simulink model "House_model"  (R2016b)
settings: Solver=VariableStepAuto  StartTime=0.0  StopTime=inf  RelTol=1e-3
settings Model: Creator=isabelle  LastModifiedBy=Josefine

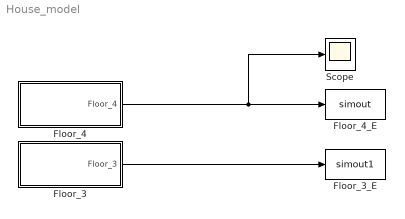
== system House_model ==
  Floor_3 : Subsystem
  Floor_3_E : ToWorkspace  VariableName=simout1  SaveFormat=Timeseries  SampleTime=-1
  Floor_4 : Subsystem
  Floor_4_E : ToWorkspace  VariableName=simout  SaveFormat=Timeseries  SampleTime=-1
  Scope : Scope
  wires:
  Floor_4/1(Floor_4) -> Scope/1, Floor_4_E/1
  Floor_3/1(Floor_3) -> Floor_3_E/1

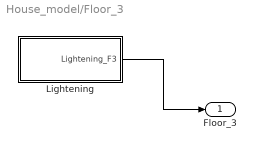
== system House_model/Floor_3 ==
  Lightening : Subsystem
  Floor_3 : Outport
  wires:
  Lightening/1(Lightening_F3) -> Floor_3/1

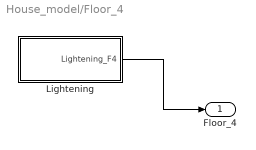
== system House_model/Floor_4 ==
  Lightening : Subsystem
  Floor_4 : Outport
  wires:
  Lightening/1(Lightening_F4) -> Floor_4/1

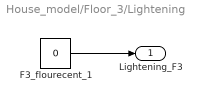
== system House_model/Floor_3/Lightening ==
  F3_flourecent_1 : Constant  Value=0
  Lightening_F3 : Outport
  wires:
  F3_flourecent_1/1 -> Lightening_F3/1

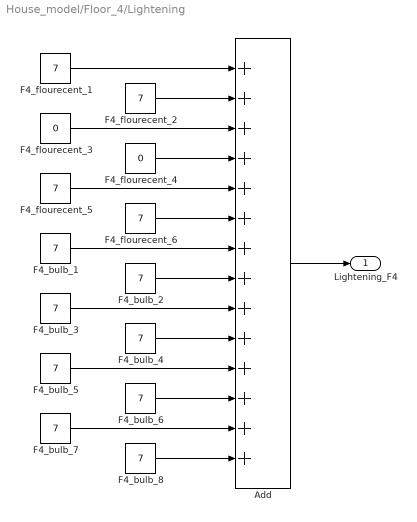
== system House_model/Floor_4/Lightening ==
  Add : Sum  Inputs=14
  F4_bulb_{1..8} (8 alike) : Constant  Value=7
  F4_flourecent_{1..2,5..6} (4 alike) : Constant  Value=7
  F4_flourecent_3 : Constant  Value=0
  F4_flourecent_4 : Constant  Value=0
  Lightening_F4 : Outport
  wires:
  F4_flourecent_1/1 -> Add/1
  F4_flourecent_2/1 -> Add/2
  F4_flourecent_3/1 -> Add/3
  F4_flourecent_4/1 -> Add/4
  F4_flourecent_5/1 -> Add/5
  F4_bulb_1/1 -> Add/7
  F4_bulb_2/1 -> Add/8
  F4_bulb_3/1 -> Add/9
  F4_bulb_4/1 -> Add/10
  F4_bulb_5/1 -> Add/11
  F4_flourecent_6/1 -> Add/6
  F4_bulb_7/1 -> Add/13
  F4_bulb_8/1 -> Add/14
  F4_bulb_6/1 -> Add/12
  Add/1 -> Lightening_F4/1
